simulink model "angular_rates_controller"  (R2019b)
settings: Solver=ode45  StartTime=0.0  StopTime=1  RelTol=1e-3  EnableMultiTasking=on
InitFcn:
  | % clear
  | clear, close all, clc
  | 
  | % load model parameters
  | load model_parameters
  | 
  | % save controller_data_rotation_dynamics K_I_RD K_f_RD
  | load controller_data
  | 
  | % initial state
  | V0 = [0.6; -0.7; 0.8];
StopFcn:
  | % draw graphics
  | angular_rates_controller_draw_graphics
undefined symbols (not defined in the file): K_f_RD, K_I_RD
settings Model: Creator=Eduardo  LastModifiedBy=bhisma
settings DataIOCC: LimitDataPoints=on  SaveFormat=Array  SignalLoggingSaveFormat=ModelDataLogs  ReturnWorkspaceOutputs=off
settings OptimizationCC: LifeSpan=inf
settings DebuggingCC: SolverPrmCheckMsg=warning  MultiTaskDSMMsg=warning  MultiTaskCondExecSysMsg=none  SFUnexpectedBacktrackingDiag=warning  SFNoUnconditionalDefaultTransitionDiag=warning  SFExecutionAtInitializationDiag=none  ArithmeticOperatorsInVariantConditions=warning
settings HardwareCC: ProdBitPerPointer=32  ProdBitPerSizeT=32  ProdBitPerPtrDiffT=32  ProdLargestAtomicFloat=None  ProdIntDivRoundTo=Undefined  ProdEndianess=Unspecified  ProdWordSize=32  ProdHWDeviceType=32-bit Generic
settings ModelReferenceCC: PropagateSignalLabelsOutOfModel=off
settings SFSimCC: SimUseLocalCustomCode=off  CustomCodeUndefinedFunction=UseInterfaceOnly
settings RTWCC: RTWUseLocalCustomCode=off
settings CodeAppCC: StateflowObjectComments=on
settings GRTTargetCC: TargetLangStandard=C89/C90 (ANSI)  GeneratePreprocessorConditionals=Disable all
settings ConfigComp: CovMetricSettings=dw  CovHtmlReporting=on  CovSaveCumulativeToWorkspaceVar=on  CovSaveSingleToWorkspaceVar=on  CovExternalEMLEnable=off

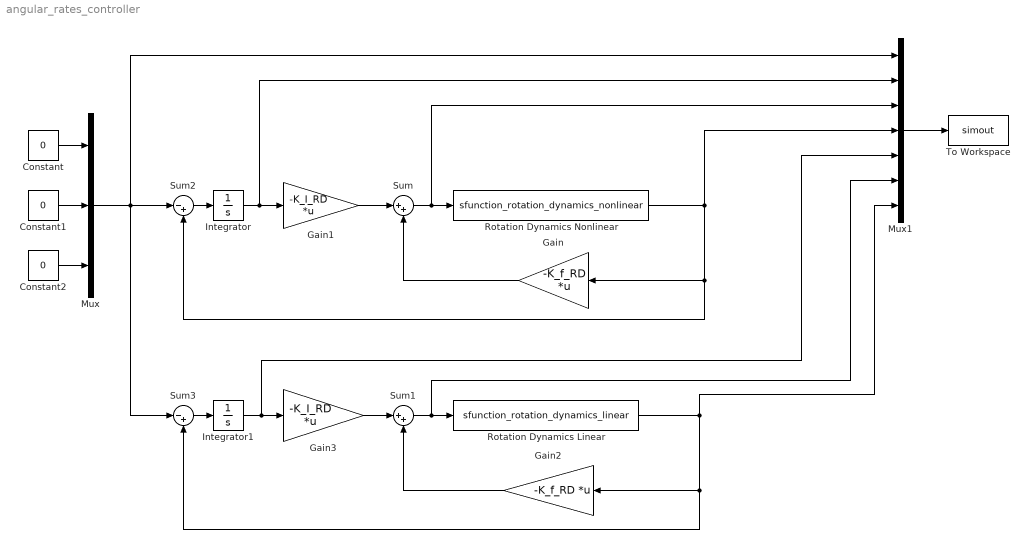
== system angular_rates_controller ==
  Constant : Constant  Value=0
  Constant1 : Constant  Value=0
  Constant2 : Constant  Value=0
  Gain : Gain  Gain=-K_f_RD  Multiplication=Matrix(K*u)
  Gain1 : Gain  Gain=-K_I_RD  Multiplication=Matrix(K*u)
  Gain2 : Gain  Gain=-K_f_RD  Multiplication=Matrix(K*u)
  Gain3 : Gain  Gain=-K_I_RD  Multiplication=Matrix(K*u)
  Integrator : Integrator  InitialCondition=[0 0 0]
  Integrator1 : Integrator  InitialCondition=[0;0;0]
  Mux : Mux  Inputs=3
  Mux1 : Mux  Inputs=7
  Rotation Dynamics Linear : S-Function  FunctionName=sfunction_rotation_dynamics_linear  Parameters=V0, Jx, Jy, Jz  SFunctionDeploymentMode=off  EnableBusSupport=off
  Rotation Dynamics Nonlinear : S-Function  FunctionName=sfunction_rotation_dynamics_nonlinear  Parameters=V0, Jx, Jy, Jz  SFunctionDeploymentMode=off  EnableBusSupport=off
  Sum : Sum  Inputs=|++
  Sum1 : Sum  Inputs=|++
  Sum2 : Sum  Inputs=|-+
  Sum3 : Sum  Inputs=|-+
  To Workspace : ToWorkspace  VariableName=simout  SaveFormat=Timeseries  SampleTime=-1
  wires:
  Sum/1 -> Mux1/3, Rotation Dynamics Nonlinear/1
  Gain/1 -> Sum/2
  Constant1/1 -> Mux/2
  Constant/1 -> Mux/1
  Constant2/1 -> Mux/3
  Sum1/1 -> Mux1/6, Rotation Dynamics Linear/1
  Gain2/1 -> Sum1/2
  Mux1/1 -> To Workspace/1
  Mux/1 -> Mux1/1, Sum3/1, Sum2/1
  Rotation Dynamics Nonlinear/1 -> Mux1/4, Sum2/2, Gain/1
  Rotation Dynamics Linear/1 -> Mux1/7, Sum3/2, Gain2/1
  Sum3/1 -> Integrator1/1
  Gain3/1 -> Sum1/1
  Sum2/1 -> Integrator/1
  Integrator/1 -> Gain1/1, Mux1/2
  Gain1/1 -> Sum/1
  Integrator1/1 -> Gain3/1, Mux1/5
